simulink model "Arduino_pid_program"  (R2017b)
settings: Solver=FixedStepDiscrete  StartTime=0.0  StopTime=Inf  RelTol=1e-3  EnableMultiTasking=on
values from neighbouring files (symbols this model uses):
  Kb = 0.01    [config.m]
  Kd = 0    [config.m]
  Ki = 0.01    [config.m]
  Kp = 0.1    [config.m]
  N = 0    [config.m]
undefined symbols (not defined in the file or in its folder): DiscIntNeverNeededParam
libraries: arduinolib x4
settings Model: ExtModeTrigDuration=2  Creator=yecheng  LastModifiedBy=Alexander
settings DataIOCC: LimitDataPoints=on  SaveFormat=Array
settings OptimizationCC: PassReuseOutputArgsAs=Individual arguments  MaxStackSize=64
settings DebuggingCC: UnderspecifiedInitializationDetection=Classic  MergeDetectMultiDrivingBlocksExec=none  ParameterTunabilityLossMsg=error  SFUnexpectedBacktrackingDiag=warning  SFNoUnconditionalDefaultTransitionDiag=warning  SFExecutionAtInitializationDiag=none
settings HardwareCC: ProdBitPerInt=16  ProdBitPerPointer=16  ProdBitPerSizeT=16  ProdBitPerPtrDiffT=16  ProdLargestAtomicFloat=None  ProdWordSize=8  ProdHWDeviceType=Atmel->AVR
settings ModelReferenceCC: PropagateSignalLabelsOutOfModel=off
settings SFSimCC: MATLABDynamicMemAlloc=off
settings RTWCC: SystemTargetFile=ert.tlc  HardwareBoard=Arduino Mega 2560  TLCOptions=-aInlineSetEventsForThisBaseRateFcn=TLC_FALSE -aSuppressMultiTaskScheduler=TLC_FALSE -aRateBasedStepFcn=1  TemplateMakefile=ert_default_tmf  GenerateReport=on  RTWVerbose=off  Toolchain=Arduino AVR  BuildConfiguration=Faster Runs  IncludeHyperlinkInReport=on  LaunchReport=on  GenerateTraceInfo=on  GenerateTraceReport=on  GenerateTraceReportSl=on  GenerateTraceReportSf=on  GenerateTraceReportEml=on
settings CodeAppCC: ForceParamTrailComments=on  IgnoreCustomStorageClasses=off  OperatorAnnotations=on  SimulinkDataObjDesc=on  SFDataObjDesc=on  InsertBlockDesc=on
settings ERTTargetCC: SupportContinuousTime=on  SupportVariableSizeSignals=on
settings ConfigComp: CovMetricSettings=dw  CovHtmlReporting=on  CovSaveCumulativeToWorkspaceVar=on  CovSaveSingleToWorkspaceVar=on  CovExternalEMLEnable=off  CovSFcnEnable=off

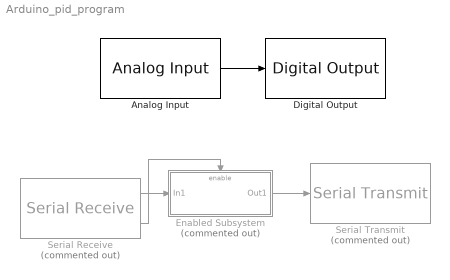
== system Arduino_pid_program ==
  Analog Input : arduinolib/Analog Input  pinNumber=4  sampleTime=1  blockPlatform=arduino
  Digital Output : arduinolib/Digital Output  pinNumber=9  blockPlatform=arduino
  Enabled Subsystem : Subsystem  Commented=on  TreatAsAtomicUnit=on
  Serial Receive : arduinolib/Serial Receive  Commented=on  isARMArch=off  portNumber=0  DataType=int32  Datalength=1  SampleTime=0.01  showOutStatus=on  blockPlatform=arduino
      settings: SourceProductName=Simulink Support Package for Arduino Hardware  SourceProductBaseCode=ARDUINO
  Serial Transmit : arduinolib/Serial Transmit  Commented=on  portNumber=0  sendmode=write  sendformat=Decimal  floatprecision=2  blockPlatform=arduino
      settings: SourceProductName=Simulink Support Package for Arduino Hardware
  wires:
  Enabled Subsystem/1(Out1) -> Serial Transmit/1
  Serial Receive/1 -> Enabled Subsystem/1(In1)
  Serial Receive/2 -> Enabled Subsystem/Enable
  Analog Input/1 -> Digital Output/1

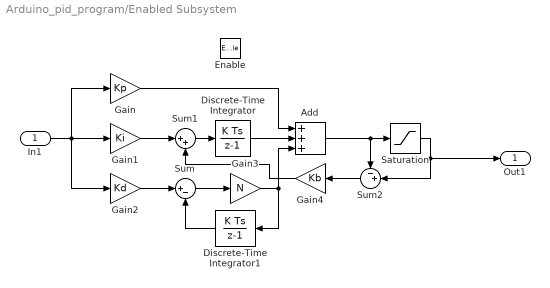
== system Arduino_pid_program/Enabled Subsystem ==
  In1 : Inport  OutDataTypeStr=int32
  Enable : EnablePort
  Add : Sum  Inputs=3
  Discrete-Time Integrator : DiscreteIntegrator  gainval=1  InitialConditionSetting=State (most efficient)  SampleTime=-1  ICPrevOutput=DiscIntNeverNeededParam  ICPrevScaledInput=DiscIntNeverNeededParam
  Discrete-Time Integrator1 : DiscreteIntegrator  gainval=1  InitialConditionSetting=State (most efficient)  SampleTime=-1  ICPrevOutput=DiscIntNeverNeededParam  ICPrevScaledInput=DiscIntNeverNeededParam
  Gain : Gain  Gain=Kp
  Gain1 : Gain  Gain=Ki
  Gain2 : Gain  Gain=Kd
  Gain3 : Gain  Gain=N  OutDataTypeStr=int32
  Gain4 : Gain  Gain=Kb
  Saturation : Saturate  UpperLimit=100000  LowerLimit=-100000  OutDataTypeStr=int32
  Sum : Sum  Inputs=|+-
  Sum1 : Sum  Inputs=|++  OutDataTypeStr=int32
  Sum2 : Sum  Inputs=-+|
  Out1 : Outport
  wires:
  Saturation/1 -> Sum2/2, Out1/1
  Add/1 -> Saturation/1, Sum2/1
  Sum/1 -> Gain3/1
  Gain2/1 -> Sum/1
  Discrete-Time Integrator/1 -> Add/2
  Sum2/1 -> Gain4/1
  Sum1/1 -> Discrete-Time Integrator/1
  Gain1/1 -> Sum1/1
  Gain4/1 -> Sum1/2
  Discrete-Time Integrator1/1 -> Sum/2
  In1/1 -> Gain/1, Gain2/1, Gain1/1
  Gain3/1 -> Discrete-Time Integrator1/1, Add/3
  Gain/1 -> Add/1
